simulink model "YCrCb_Color_Component_ManualThresholding"  (R2016a)
settings: Solver=VariableStepAuto  StartTime=0.0  StopTime=10.0  RelTol=1e-3
undefined symbols (not defined in the file): Rec, SDTV
libraries: visionstatistics x6, visionconversions x3, visionsinks x3, visionsources x1
settings Model: Creator=YASARA  LastModifiedBy=YASARA

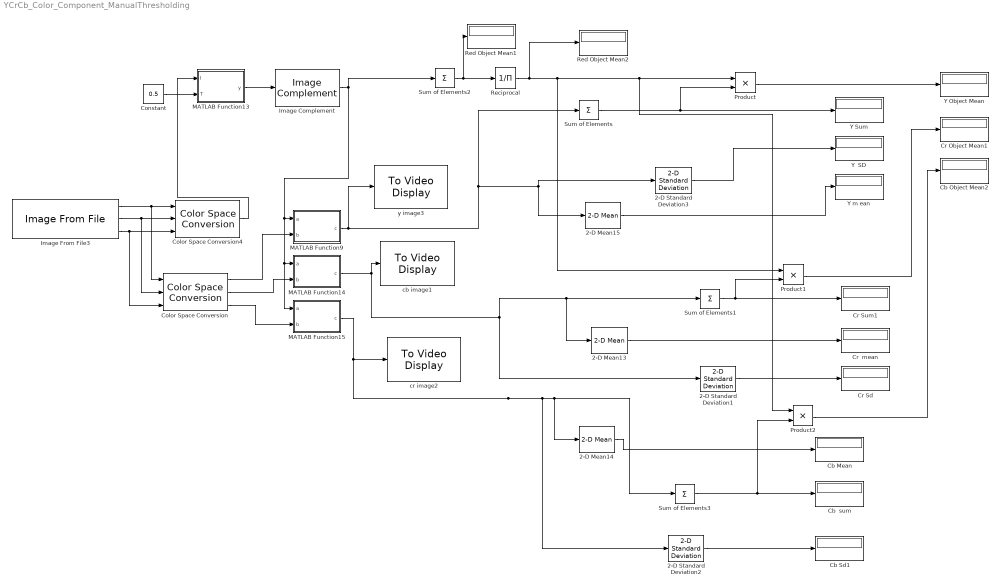
== system YCrCb_Color_Component_ManualThresholding ==
  2-D Mean13 : visionstatistics/2-D Mean  run=off  reset_popup=None  directionMode=Entire input  dimension=1  treatSBRowAsCol=on  roiEnable=off  roiType=Rectangles  roiPortion=Entire ROI  roiOutput=Individual statistics for each ROI  roiFlag=off  outputDataTypeStr=Inherit: Same as accumulator  outputLastDataTypeStr=Inherit: Same as accumulator  outputMin=[]  outputMax=[]  accumMode=Binary point scaling  accumWordLength=32  accumFracLength=0  accumDataTypeStr=fixdt([],32,0)  accumLastDataTypeStr=fixdt([],32,0)  roundingMode=Floor  overflowMode=off
  2-D Mean14 : visionstatistics/2-D Mean  run=off  reset_popup=None  directionMode=Entire input  dimension=1  treatSBRowAsCol=on  roiEnable=off  roiType=Rectangles  roiPortion=Entire ROI  roiOutput=Individual statistics for each ROI  roiFlag=off  outputDataTypeStr=Inherit: Same as accumulator  outputLastDataTypeStr=Inherit: Same as accumulator  outputMin=[]  outputMax=[]  accumMode=Binary point scaling  accumWordLength=32  accumFracLength=0  accumDataTypeStr=fixdt([],32,0)  accumLastDataTypeStr=fixdt([],32,0)  roundingMode=Floor  overflowMode=off
  2-D Mean15 : visionstatistics/2-D Mean  run=off  reset_popup=None  directionMode=Entire input  dimension=1  treatSBRowAsCol=on  roiEnable=off  roiType=Rectangles  roiPortion=Entire ROI  roiOutput=Individual statistics for each ROI  roiFlag=off  outputDataTypeStr=Inherit: Same as accumulator  outputLastDataTypeStr=Inherit: Same as accumulator  outputMin=[]  outputMax=[]  accumMode=Binary point scaling  accumWordLength=32  accumFracLength=0  accumDataTypeStr=fixdt([],32,0)  accumLastDataTypeStr=fixdt([],32,0)  roundingMode=Floor  overflowMode=off
  2-D Standard Deviation1 : visionstatistics/2-D Standard Deviation  run=off  reset_popup=None  directionMode=Entire input  dimension=1  treatSBRowAsCol=on  roiEnable=off  roiType=Rectangles  roiPortion=Entire ROI  roiOutput=Individual statistics for each ROI  roiFlag=off
  2-D Standard Deviation2 : visionstatistics/2-D Standard Deviation  run=off  reset_popup=None  directionMode=Entire input  dimension=1  treatSBRowAsCol=on  roiEnable=off  roiType=Rectangles  roiPortion=Entire ROI  roiOutput=Individual statistics for each ROI  roiFlag=off
  2-D Standard Deviation3 : visionstatistics/2-D Standard Deviation  run=off  reset_popup=None  directionMode=Entire input  dimension=1  treatSBRowAsCol=on  roiEnable=off  roiType=Rectangles  roiPortion=Entire ROI  roiOutput=Individual statistics for each ROI  roiFlag=off
  Cb  sum : Display
  Cb Mean : Display
  Cb Object Mean2 : Display
  Cb Sd1 : Display
  Color Space Conversion : visionconversions/Color Space  Conversion  conversion=Obsolete  conversionActive=R'G'B' to Y'CbCr  wp_str=D65  rec=Rec. 601 (SDTV)  sys=1125/60/2:1  imagePorts=Separate color signals
  Color Space Conversion4 : visionconversions/Color Space  Conversion  conversion=Obsolete  conversionActive=R'G'B' to intensity  wp_str=D65  rec=Rec. 601 (SDTV)  sys=1125/60/2:1  imagePorts=Separate color signals
  Constant : Constant  Value=0.5  SampleTime=1
  Cr  mean : Display
  Cr Object Mean1 : Display
  Cr Sd : Display
  Cr Sum1 : Display
  Image Complement : visionconversions/Image Complement
  Image From File3 : visionsources/Image From File  Tag=vipblks_nd  FileName=C:\Users\YASARA\Desktop\FRY_Docu\tea\teaxb.jpg  imagePorts=Separate color signals  Ts=1  ImageDataType=double  Signed=on  WordLength=16  sdImageDataType=uint(8)  FractionLengthMode=User-defined  FractionLength=15  OutPortLabels=R|G|B
  MATLAB Function13 : MATLAB Function  TreatAsAtomicUnit=on
  MATLAB Function14 : MATLAB Function  TreatAsAtomicUnit=on
  MATLAB Function15 : MATLAB Function  TreatAsAtomicUnit=on
  MATLAB Function9 : MATLAB Function  TreatAsAtomicUnit=on
  Product : Product
  Product1 : Product
  Product2 : Product
  Reciprocal : Product  Inputs=/  OutDataTypeStr=double  SaturateOnIntegerOverflow=on  RndMeth=Zero
  Red Object Mean1 : Display
  Red Object Mean2 : Display
  Sum of Elements{,1..3} (4 alike) : Sum  Inputs=+
  Y  SD : Display
  Y Object Mean : Display
  Y Sum : Display
  Y m ean : Display
  cb image1 : visionsinks/To Video Display  windowSizeMode=Normal  openAtMdlStart=on  fullScreen=off  videoWindowX=252  videoWindowY=213  saveWindowSize=off  videoWindowWidth=512  videoWindowHeight=384  inputColorFormat=RGB  inputType=Obsolete  imagePorts=One multidimensional signal  OutputDevice=On-screen video monitor  dataOrg=Column-major  isWindowOpen=off
  cr image2 : visionsinks/To Video Display  windowSizeMode=Normal  openAtMdlStart=on  fullScreen=off  videoWindowX=252  videoWindowY=213  saveWindowSize=off  videoWindowWidth=512  videoWindowHeight=384  inputColorFormat=RGB  inputType=Obsolete  imagePorts=One multidimensional signal  OutputDevice=On-screen video monitor  dataOrg=Column-major  isWindowOpen=off
  y image3 : visionsinks/To Video Display  windowSizeMode=Normal  openAtMdlStart=on  fullScreen=off  videoWindowX=252  videoWindowY=213  saveWindowSize=off  videoWindowWidth=512  videoWindowHeight=384  inputColorFormat=RGB  inputType=Obsolete  imagePorts=One multidimensional signal  OutputDevice=On-screen video monitor  dataOrg=Column-major  isWindowOpen=off
  wires:
  Image From File3/1 -> Color Space Conversion/1, Color Space Conversion4/1
  Image From File3/2 -> Color Space Conversion/2, Color Space Conversion4/2
  Image From File3/3 -> Color Space Conversion/3, Color Space Conversion4/3
  MATLAB Function13/1(y) -> Image Complement/1
  Color Space Conversion4/1 -> MATLAB Function13/1(I)
  2-D Mean15/1 -> Y m ean/1
  2-D Mean13/1 -> Cr  mean/1
  Sum of Elements/1 -> Product/2, Y Sum/1
  MATLAB Function9/1(c) -> y image3/1, Sum of Elements/1, 2-D Mean15/1, 2-D Standard Deviation3/1
  2-D Standard Deviation3/1 -> Y  SD/1
  2-D Standard Deviation1/1 -> Cr Sd/1
  MATLAB Function14/1(c) -> cb image1/1, 2-D Mean13/1, Sum of Elements1/1, 2-D Standard Deviation1/1
  Sum of Elements3/1 -> Product2/2, Cb  sum/1
  2-D Standard Deviation2/1 -> Cb Sd1/1
  MATLAB Function15/1(c) -> 2-D Standard Deviation2/1, 2-D Mean14/1, Sum of Elements3/1, cr image2/1
  Constant/1 -> MATLAB Function13/2(T)
  Sum of Elements2/1 -> Red Object Mean1/1, Reciprocal/1
  Product/1 -> Y Object Mean/1
  Sum of Elements1/1 -> Product1/2, Cr Sum1/1
  Product1/1 -> Cr Object Mean1/1
  2-D Mean14/1 -> Cb Mean/1
  Product2/1 -> Cb Object Mean2/1
  Reciprocal/1 -> Red Object Mean2/1, Product2/1, Product/1, Product1/1
  Image Complement/1 -> MATLAB Function15/1(a), MATLAB Function14/1(a), MATLAB Function9/1(a), Sum of Elements2/1
  Color Space Conversion/1 -> MATLAB Function9/2(b)
  Color Space Conversion/2 -> MATLAB Function14/2(b)
  Color Space Conversion/3 -> MATLAB Function15/2(b)

== matlab function YCrCb_Color_Component_ManualThresholding/MATLAB Function14 ==
  data: a input; b input; c output
function c = fcn(a,b)
%#codegen
c=a.*b;
return

== matlab function YCrCb_Color_Component_ManualThresholding/MATLAB Function13 ==
  data: I input; y output; T input
function y = fcn(I,T)
%#codegen
BW = imbinarize(I,T);
y = BW;

== matlab function YCrCb_Color_Component_ManualThresholding/MATLAB Function15 ==
  data: a input; b input; c output
function c = fcn(a,b)
%#codegen
c=a.*b;
return

== matlab function YCrCb_Color_Component_ManualThresholding/MATLAB Function9 ==
  data: a input; b input; c output
function c = fcn(a,b)
%#codegen
c=a.*b;
return
